simulink model "LimitCycle_EncoderTest"  (R2022b)
settings: Solver=FixedStepAuto  StartTime=0.0  StopTime=inf  RelTol=1e-3  EnableMultiTasking=on
model workspace (MAT data in the model file):
  sampleRate = 0.01
libraries: arduinomotorcarrierlib x3, eeGeneralControl x3, arduinolib x2, mkrmotorcarrierlib x1, simulink x1
settings Model: ExtModeTrigDuration=2  Creator=bkhusain  LastModifiedBy=arkad
settings SolverCC: AlgebraicLoopSolver=TrustRegion
settings DataIOCC: ReturnWorkspaceOutputs=off
settings OptimizationCC: EnhancedBackFolding=on  PassReuseOutputArgsThreshold=0  MaxStackSize=64  OptimizeBlockOrder=speed  DifferentSizesBufferReuse=on  OptimizationCustomize=off
settings DebuggingCC: ParameterOverflowMsg=none  ParameterUnderflowMsg=error  ParameterPrecisionLossMsg=none  ParameterTunabilityLossMsg=error  UnconnectedInputMsg=warning  UnconnectedOutputMsg=warning  UnconnectedLineMsg=warning  SFMachineParentedDataDiag=warning
settings HardwareCC: ProdBitPerPointer=32  ProdBitPerSizeT=32  ProdBitPerPtrDiffT=32  ProdLargestAtomicInteger=Long  ProdLargestAtomicFloat=Double  ProdWordSize=32  ProdHWDeviceType=ARM Compatible->ARM Cortex
settings ModelReferenceCC: EnableRefExpFcnMdlSchedulingChecks=on
settings SFSimCC: MATLABDynamicMemAlloc=off
settings RTWCC: Description=Embedded Coder  SystemTargetFile=ert.tlc  HardwareBoard=Arduino MKRZero  TLCOptions=-aInlineSetEventsForThisBaseRateFcn=TLC_FALSE -aSuppressMultiTaskScheduler=TLC_FALSE -aRateBasedStepFcn=1  TemplateMakefile=ert_default_tmf  Toolchain=Arduino ARM  BuildConfiguration=Faster Runs  DLArmComputeVersion=19.05
settings CodeAppCC: ForceParamTrailComments=on  OperatorAnnotations=on
settings ERTTargetCC: ERTCustomFileBanners=off  SupportContinuousTime=on  SupportNonInlinedSFcns=on  RemoveResetFunc=off  SupportVariableSizeSignals=on  ModelStepFunctionPrototypeControlCompliant=off  ExtModeTransport=3  ExtModeStaticAlloc=on  ExtModeAutomaticAllocSize=off  ExtModeStaticAllocSize=8192  ExtModeMexFile=ext_xcp  ExtModeIntrfLevel=Level2 - Open

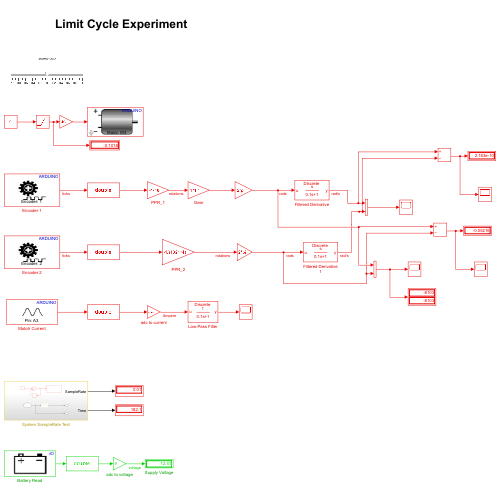
[thumbnail: Simulink's stored preview of the top-level diagram]
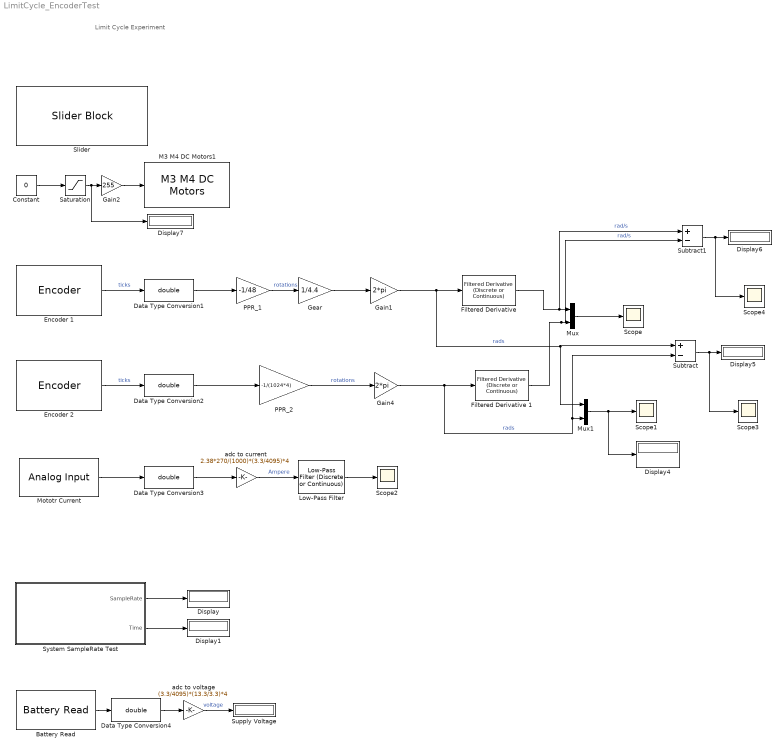
== system LimitCycle_EncoderTest ==
  note: Limit Cycle Experiment
  Battery Read : arduinomotorcarrierlib/Battery Read  SlaveAddress=uint8( hex2dec( '66' ) )  blockPlatform=ARDUINO  SampleTime=0.1
  Constant : Constant  Value=0  SampleTime=sampleRate
  Data Type Conversion{1..4} (4 alike) : DataTypeConversion  OutDataTypeStr=double  SaturateOnIntegerOverflow=off  RndMeth=Floor
  Display{,1,4..7} (6 alike) : Display
      Display7 settings: Decimation=3
  Encoder 1 : arduinomotorcarrierlib/Encoder  SlaveAddress=uint8( hex2dec( '66' ) )  blockPlatform=ARDUINO  Encoder=1  ShowSpeed=off  ResetOption=on  SampleTime=sampleRate
  Encoder 2 : arduinomotorcarrierlib/Encoder  SlaveAddress=uint8( hex2dec( '66' ) )  blockPlatform=ARDUINO  Encoder=2  ShowSpeed=off  ResetOption=on  SampleTime=sampleRate
  "Filtered Derivative " : eeGeneralControl/Filtered Derivative (Discrete or Continuous)  K=1  T=0.1  B=inf  A=-inf  minRatio=10  init_option=Inherited from block input  x0=0  Ts=-1
  Filtered Derivative 1 : eeGeneralControl/Filtered Derivative (Discrete or Continuous)  K=1  T=0.1  B=inf  A=-inf  minRatio=10  init_option=Inherited from block input  x0=0  Ts=-1
  Gain1 : Gain  Gain=2*pi
  Gain2 : Gain  Gain=255
  Gain4 : Gain  Gain=2*pi
  Gear : Gain  Gain=1/4.4
  Low-Pass Filter : eeGeneralControl/Low-Pass Filter (Discrete or Continuous)  K=1  T=0.1  B=inf  A=-inf  init_option=Inherited from block input  x0=0  Ts=-1
  M3 M4 DC Motors1 : mkrmotorcarrierlib/M3 M4 DC Motors  MotorNumber=M3  forwardPinNumber=3  reversePinNumber=2
  Mototr Current : arduinolib/Analog Input  pinNumber=3  ReadResultsOnly=off  ConversionTriggerSource=Software  ExternalTriggerType=uint32( 0 )  OutputDataType=uint16  EnableConversionCompleteNotify=off  EnableOuputStatus=off  SampleTime=sampleRate  blockPlatform=arduino
  Mux : Mux  Inputs=2
  Mux1 : Mux  Inputs=2
  PPR_1 : Gain  Gain=-1/48
  PPR_2 : Gain  Gain=-1/(1024*4)
  Saturation : Saturate  UpperLimit=1  LowerLimit=-1
  Scope{,1..4} (5 alike) : Scope
  Slider : SliderBlock  ScaleMin=-1  ScaleMax=1
  Subtract : Sum  Inputs=+-
  Subtract1 : Sum  Inputs=+-
  Supply Voltage : Display
  System SampleRate Test : Subsystem
  adc to current : Gain  Gain=2.38*270/(1000)*(3.3/4095)*4
  adc to voltage : Gain  Gain=(3.3/4095)*(13.3/3.3)*4
  wires:
  PPR_1/1 -> Gear/1  "rotations"
  Gain1/1 -> Mux1/1, Subtract/1, "Filtered Derivative "/1  "rads"
  Encoder 1/1 -> Data Type Conversion1/1  "ticks"
  Gain2/1 -> M3 M4 DC Motors1/1
  Constant/1 -> Saturation/1
  Saturation/1 -> Display7/1, Gain2/1
  "Filtered Derivative "/1 -> Subtract1/1, Mux/1  "rad/s"
  Mux/1 -> Scope/1
  Filtered Derivative 1/1 -> Subtract1/2, Mux/2  "rad/s"
  Gain4/1 -> Subtract/2, Mux1/2, Filtered Derivative 1/1  "rads"
  Data Type Conversion2/1 -> PPR_2/1
  PPR_2/1 -> Gain4/1  "rotations"
  Encoder 2/1 -> Data Type Conversion2/1  "ticks"
  Mux1/1 -> Display4/1, Scope1/1
  Mototr Current/1 -> Data Type Conversion3/1
  System SampleRate Test/1(SampleRate) -> Display/1
  System SampleRate Test/2(Time) -> Display1/1
  Battery Read/1 -> Data Type Conversion4/1
  adc to voltage/1 -> Supply Voltage/1  "voltage"
  adc to current/1 -> Low-Pass Filter/1  "Ampere"
  Low-Pass Filter/1 -> Scope2/1
  Data Type Conversion3/1 -> adc to current/1
  Gear/1 -> Gain1/1
  Data Type Conversion1/1 -> PPR_1/1
  Subtract/1 -> Scope3/1, Display5/1
  Data Type Conversion4/1 -> adc to voltage/1
  Subtract1/1 -> Scope4/1, Display6/1

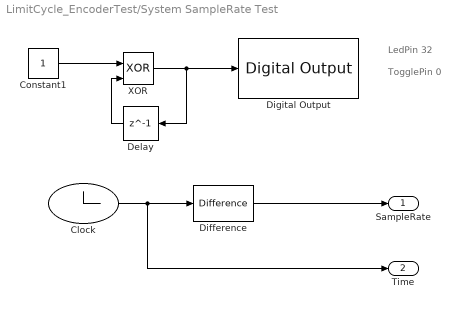
== system LimitCycle_EncoderTest/System SampleRate Test ==
  note: LedPin 32
  note: TogglePin 0
  Clock : Clock
      settings: Decimation=3
  Constant1 : Constant  SampleTime=sampleRate
  Delay : Delay  DelayLength=1  InitialCondition=0  SampleTime=sampleRate
  Difference : simulink/Quick Insert/Discrete/Difference  ICPrevInput=0.0  OutMin=[]  OutMax=[]  OutDataType=fixdt(1, 16)  OutScaling=2^-10  DoSatur=off
  Digital Output : arduinolib/Digital Output  pinNumber=0  Direction=output  blockPlatform=arduino
  XOR : Logic  Operator=XOR  IconShape=distinctive  AllPortsSameDT=off  OutDataTypeStr=boolean
  SampleRate : Outport
  Time : Outport  Port=2
  wires:
  XOR/1 -> Delay/1, Digital Output/1
  Constant1/1 -> XOR/1
  Delay/1 -> XOR/2
  Clock/1 -> Time/1, Difference/1
  Difference/1 -> SampleRate/1
